simulink model "Model"  (R2020b)
settings: Solver=VariableStepAuto  StartTime=0.0  StopTime=10.0  RelTol=1e-3
values from neighbouring files (symbols this model uses):
  body = block.DialogPrm(2).Data    [sfun_balrob_long_dyn.m]
  ms22g = 1/g    (= 0.101936799185)    [LoadParameters.m]
  Ts = 1e-2    (= 0.01)    [LoadParameters.m]
undefined symbols (not defined in the file or in its folder): drv, sens, ua2tau
settings Model: Creator=Utente  LastModifiedBy=Utente

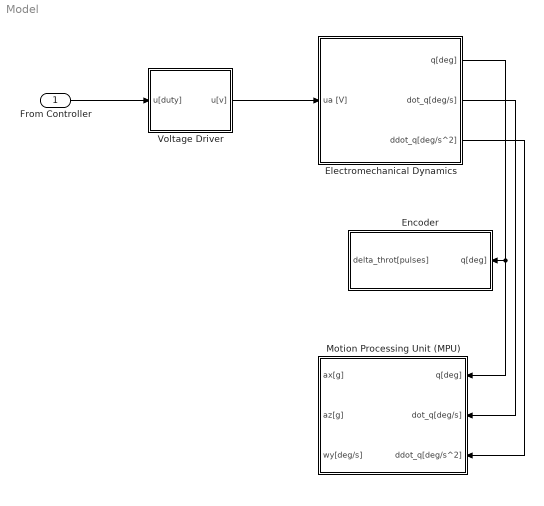
== system Model ==
  From Controller : Inport
  Electromechanical Dynamics : Subsystem
  Encoder : Subsystem
  Motion Processing Unit (MPU) : Subsystem
  Voltage Driver : Subsystem
  wires:
  Voltage Driver/1(u[v]) -> Electromechanical Dynamics/1(ua [V])
  From Controller/1 -> Voltage Driver/1(u[duty])
  Electromechanical Dynamics/1(q[deg]) -> Motion Processing Unit (MPU)/1(q[deg]), Encoder/1(q[deg])
  Electromechanical Dynamics/2(dot_q[deg/s]) -> Motion Processing Unit (MPU)/2(dot_q[deg/s])
  Electromechanical Dynamics/3(ddot_q[deg/s^2]) -> Motion Processing Unit (MPU)/3(ddot_q[deg/s^2])

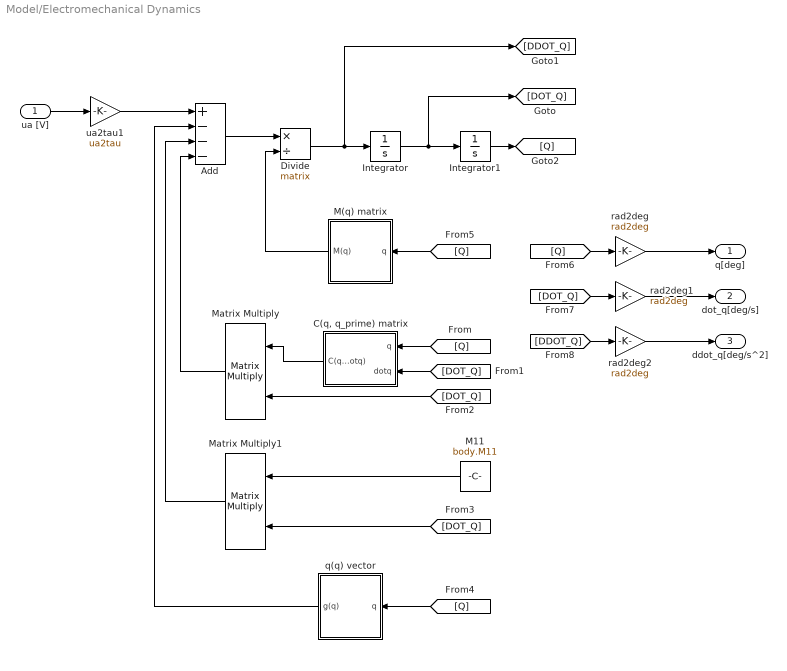
== system Model/Electromechanical Dynamics ==
  ua [V] : Inport
  Add : Sum  Inputs=+---
  "C(q, q_prime) matrix" : Subsystem
  Divide : Product  Inputs=*/  Multiplication=Matrix(*)
  Integrator : Integrator
  Integrator1 : Integrator
  M(q) matrix : Subsystem
  M11 : Constant  Value=body.M11
  Matrix Multiply : Product  Multiplication=Matrix(*)
  Matrix Multiply1 : Product  Multiplication=Matrix(*)
  q(q) vector : Subsystem
  rad2deg : Gain  Gain=rad2deg
  rad2deg1 : Gain  Gain=rad2deg
  rad2deg2 : Gain  Gain=rad2deg
  ua2tau1 : Gain  Gain=ua2tau
  q[deg] : Outport
  dot_q[deg/s] : Outport  Port=2
  ddot_q[deg/s^2] : Outport  Port=3
  wires:
  Add/1 -> Divide/1
  Integrator/1 -> [DOT_Q], Integrator1/1
  [Q] -> M(q) matrix/1(q)
  [Q] -> rad2deg/1
  Matrix Multiply1/1 -> Add/3
  rad2deg2/1 -> ddot_q[deg/s^2]/1
  M11/1 -> Matrix Multiply1/1
  rad2deg/1 -> q[deg]/1
  Integrator1/1 -> [Q]
  [DOT_Q] -> Matrix Multiply1/2
  rad2deg1/1 -> dot_q[deg/s]/1
  M(q) matrix/1(M(q)) -> Divide/2
  Matrix Multiply/1 -> Add/4
  Divide/1 -> [DDOT_Q], Integrator/1
  q(q) vector/1(g(q)) -> Add/2
  ua [V]/1 -> ua2tau1/1
  ua2tau1/1 -> Add/1
  [DOT_Q] -> rad2deg1/1
  [DOT_Q] -> Matrix Multiply/2
  [Q] -> q(q) vector/1(q)
  [DDOT_Q] -> rad2deg2/1
  [DOT_Q] -> "C(q, q_prime) matrix"/2(dotq)
  [Q] -> "C(q, q_prime) matrix"/1(q)
  "C(q, q_prime) matrix"/1("C(q, dotq)") -> Matrix Multiply/1

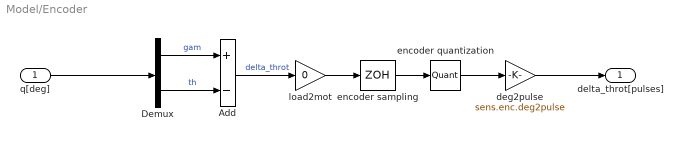
== system Model/Encoder ==
  q[deg] : Inport
  Add : Sum  Inputs=+-
  Demux : Demux  Outputs=2
  deg2pulse : Gain  Gain=sens.enc.deg2pulse
  encoder quantization : Quantizer  QuantizationInterval=sens.enc.pulse2deg
  encoder sampling : ZeroOrderHold  SampleTime=Ts
  load2mot : Gain  Gain=0
  delta_throt[pulses] : Outport
  wires:
  Add/1 -> load2mot/1  "delta_throt"
  encoder sampling/1 -> encoder quantization/1
  load2mot/1 -> encoder sampling/1
  encoder quantization/1 -> deg2pulse/1
  Demux/2 -> Add/2  "th"
  deg2pulse/1 -> delta_throt[pulses]/1
  q[deg]/1 -> Demux/1
  Demux/1 -> Add/1  "gam"

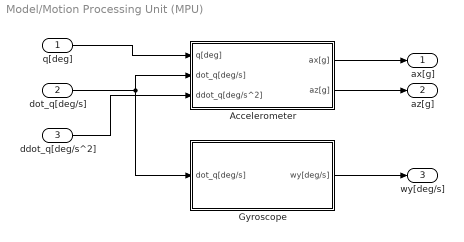
== system Model/Motion Processing Unit (MPU) ==
  q[deg] : Inport
  dot_q[deg/s] : Inport  Port=2
  ddot_q[deg/s^2] : Inport  Port=3
  Accelerometer : Subsystem
  Gyroscope : Subsystem
  ax[g] : Outport
  az[g] : Outport  Port=2
  wy[deg/s] : Outport  Port=3
  wires:
  ddot_q[deg/s^2]/1 -> Accelerometer/3(ddot_q[deg/s^2])
  Accelerometer/1(ax[g]) -> ax[g]/1
  q[deg]/1 -> Accelerometer/1("q[deg] ")
  dot_q[deg/s]/1 -> Gyroscope/1("dot_q[deg/s] "), Accelerometer/2(dot_q[deg/s])
  Gyroscope/1(wy[deg/s]) -> wy[deg/s]/1
  Accelerometer/2(az[g]) -> az[g]/1

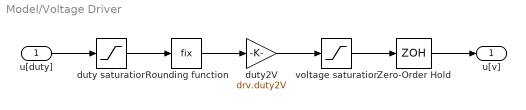
== system Model/Voltage Driver ==
  u[duty] : Inport
  Rounding function : Rounding  Operator=fix
  Zero-Order Hold : ZeroOrderHold  SampleTime=Ts
  duty saturation : Saturate  UpperLimit=drv.dutymax  LowerLimit=-drv.dutymax
  duty2V : Gain  Gain=drv.duty2V
  voltage saturation : Saturate  UpperLimit=drv.Vbus  LowerLimit=-drv.Vbus
  u[v] : Outport
  wires:
  Zero-Order Hold/1 -> u[v]/1
  u[duty]/1 -> duty saturation/1
  duty saturation/1 -> Rounding function/1
  voltage saturation/1 -> Zero-Order Hold/1
  duty2V/1 -> voltage saturation/1
  Rounding function/1 -> duty2V/1

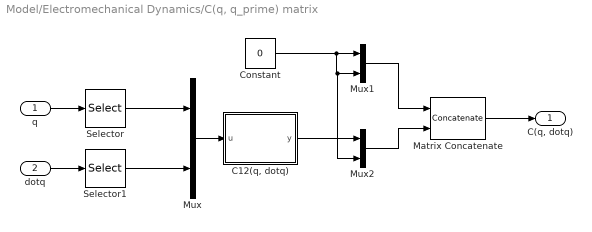
== system Model/Electromechanical Dynamics/C(q, q_prime) matrix ==
  q : Inport
  dotq : Inport  Port=2
  "C12(q, dotq)" : MATLAB Function  TreatAsAtomicUnit=on
  Constant : Constant  Value=0
  Matrix Concatenate : Concatenate  Mode=Multidimensional array  ConcatenateDimension=2
  Mux : Mux  Inputs=2
  Mux1 : Mux  Inputs=2
  Mux2 : Mux  Inputs=2
  Selector : Selector  InputPortWidth=2  IndexOptions=Index vector (dialog)  Indices=2  OutputSizes=1
  Selector1 : Selector  InputPortWidth=2  IndexOptions=Index vector (dialog)  Indices=2  OutputSizes=1
  "C(q, dotq)" : Outport
  wires:
  Constant/1 -> Mux2/2, Mux1/2, Mux1/1
  Mux/1 -> "C12(q, dotq)"/1(u)
  Mux2/1 -> Matrix Concatenate/2
  dotq/1 -> Selector1/1
  q/1 -> Selector/1
  Matrix Concatenate/1 -> "C(q, dotq)"/1
  Mux1/1 -> Matrix Concatenate/1
  Selector/1 -> Mux/1
  "C12(q, dotq)"/1(y) -> Mux2/1
  Selector1/1 -> Mux/2

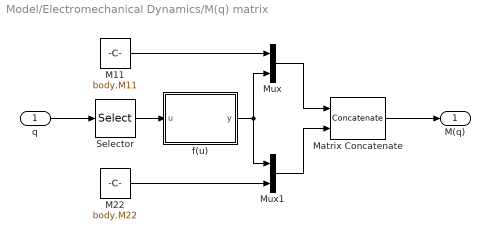
== system Model/Electromechanical Dynamics/M(q) matrix ==
  q : Inport
  M11 : Constant  Value=body.M11
  M22 : Constant  Value=body.M22
  Matrix Concatenate : Concatenate  Mode=Multidimensional array  ConcatenateDimension=2
  Mux : Mux  Inputs=2
  Mux1 : Mux  Inputs=2
  Selector : Selector  InputPortWidth=2  IndexOptions=Index vector (dialog)  Indices=2  OutputSizes=1
  f(u) : MATLAB Function  TreatAsAtomicUnit=on
  M(q) : Outport
  wires:
  Mux/1 -> Matrix Concatenate/1
  Selector/1 -> f(u)/1(u)
  M22/1 -> Mux1/2
  f(u)/1(y) -> Mux1/1, Mux/2
  q/1 -> Selector/1
  Matrix Concatenate/1 -> M(q)/1
  Mux1/1 -> Matrix Concatenate/2
  M11/1 -> Mux/1

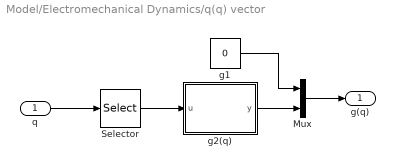
== system Model/Electromechanical Dynamics/q(q) vector ==
  q : Inport
  Mux : Mux  Inputs=2
  Selector : Selector  InputPortWidth=2  IndexOptions=Index vector (dialog)  Indices=2  OutputSizes=1
  g1 : Constant  Value=0
  g2(q) : MATLAB Function  TreatAsAtomicUnit=on
  g(q) : Outport
  wires:
  g1/1 -> Mux/1
  Mux/1 -> g(q)/1
  g2(q)/1(y) -> Mux/2
  q/1 -> Selector/1
  Selector/1 -> g2(q)/1(u)

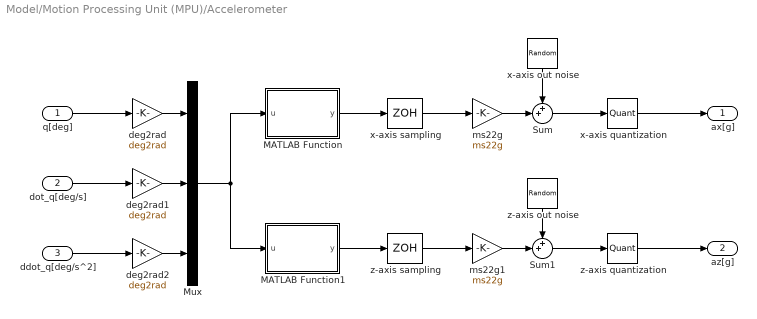
== system Model/Motion Processing Unit (MPU)/Accelerometer ==
  "q[deg] " : Inport
  dot_q[deg/s] : Inport  Port=2
  ddot_q[deg/s^2] : Inport  Port=3
  MATLAB Function : MATLAB Function  TreatAsAtomicUnit=on
  MATLAB Function1 : MATLAB Function  TreatAsAtomicUnit=on
  Mux : Mux  Inputs=3
  Sum : Sum  Inputs=++|
  Sum1 : Sum  Inputs=++|
  deg2rad : Gain  Gain=deg2rad
  deg2rad1 : Gain  Gain=deg2rad
  deg2rad2 : Gain  Gain=deg2rad
  ms22g : Gain  Gain=ms22g
  ms22g1 : Gain  Gain=ms22g
  x-axis out noise : RandomNumber  Variance=sens.mpu.acc.noisevar  SampleTime=0.1
  x-axis quantization : Quantizer  QuantizationInterval=sens.mpu.acc.LSB2g
  x-axis sampling : ZeroOrderHold  SampleTime=-1
  z-axis out noise : RandomNumber  Variance=sens.mpu.acc.noisevar  SampleTime=0.1
  z-axis quantization : Quantizer  QuantizationInterval=sens.mpu.acc.LSB2g
  z-axis sampling : ZeroOrderHold  SampleTime=-1
  ax[g] : Outport
  az[g] : Outport  Port=2
  wires:
  x-axis sampling/1 -> ms22g/1
  z-axis quantization/1 -> az[g]/1
  deg2rad1/1 -> Mux/2
  x-axis quantization/1 -> ax[g]/1
  ms22g/1 -> Sum/2
  dot_q[deg/s]/1 -> deg2rad1/1
  ms22g1/1 -> Sum1/2
  Sum/1 -> x-axis quantization/1
  Sum1/1 -> z-axis quantization/1
  z-axis out noise/1 -> Sum1/1
  z-axis sampling/1 -> ms22g1/1
  x-axis out noise/1 -> Sum/1
  MATLAB Function/1(y) -> x-axis sampling/1
  Mux/1 -> MATLAB Function/1(u), MATLAB Function1/1(u)
  MATLAB Function1/1(y) -> z-axis sampling/1
  deg2rad2/1 -> Mux/3
  ddot_q[deg/s^2]/1 -> deg2rad2/1
  deg2rad/1 -> Mux/1
  "q[deg] "/1 -> deg2rad/1

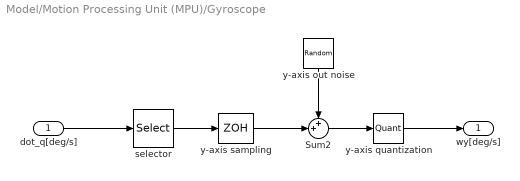
== system Model/Motion Processing Unit (MPU)/Gyroscope ==
  "dot_q[deg/s] " : Inport
  Sum2 : Sum  Inputs=++|
  selector : Selector  InputPortWidth=2  IndexOptions=Index vector (dialog)  Indices=[2]  OutputSizes=1
  y-axis out noise : RandomNumber  Variance=sens.mpu.gyro.noisevar  SampleTime=0.1
  y-axis quantization : Quantizer  QuantizationInterval=sens.mpu.gyro.LSB2g
  y-axis sampling : ZeroOrderHold  SampleTime=-1
  wy[deg/s] : Outport
  wires:
  Sum2/1 -> y-axis quantization/1
  y-axis out noise/1 -> Sum2/1
  y-axis quantization/1 -> wy[deg/s]/1
  selector/1 -> y-axis sampling/1
  y-axis sampling/1 -> Sum2/2
  "dot_q[deg/s] "/1 -> selector/1

== matlab function Model/Electromechanical Dynamics/q(q) vector/g2(q) ==
  data: u input; y output
function y = f(u)

y = 0;

== matlab function Model/Electromechanical Dynamics/C(q, q_prime) matrix/C12(q, dotq) ==
  data: u input; y output
function y = f(u)
theta = u(1,1);
theta_dot = u(2, 1);
y = -(body.m*body.zb+2*mot.rot.m*mot.rot.zb)*wheel.r*sin(theta)*theta_dot;

== matlab function Model/Motion Processing Unit (MPU)/Accelerometer/MATLAB Function ==
  data: u input; y output
function y = fcn(u)

y = u;

== matlab function Model/Motion Processing Unit (MPU)/Accelerometer/MATLAB Function1 ==
  data: u input; y output
function y = fcn(u)

y = u;

== matlab function Model/Electromechanical Dynamics/M(q) matrix/f(u) ==
  data: u input; y output
function y = f(u)
y = 2*gbox.N*(1-gbox.N)*mot.rot.Iyy+(body.m*body.zb+2*mot.rot.m*mot.rot.zb)*wheel.r*cos(u);
